simulink subsystem "Falphabeta_to_Fdq"  (R2019b)
settings: Solver=VariableStepAuto  StartTime=0.0  StopTime=10.0  RelTol=1e-3
settings Model: Creator=Nathan Petersen  LastModifiedBy=Nathan Petersen

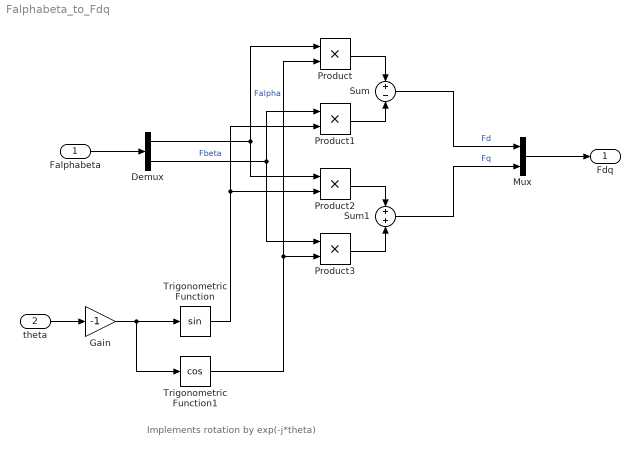
== system Falphabeta_to_Fdq ==
  note: Implements rotation by exp(-j*theta)
  Falphabeta : Inport  PortDimensions=2
  theta : Inport  Port=2  PortDimensions=1
  Demux : Demux  Outputs=2
  Gain : Gain  Gain=-1
  Mux : Mux  Inputs=2
  Product{,1..3} (4 alike) : Product
  Sum : Sum  Inputs=+-
  Sum1 : Sum
  Trigonometric Function : Trigonometry
  Trigonometric Function1 : Trigonometry  Operator=cos
  Fdq : Outport  PortDimensions=2
  wires:
  Falphabeta/1 -> Demux/1
  Product1/1 -> Sum/2
  theta/1 -> Gain/1
  Product3/1 -> Sum1/2
  Sum/1 -> Mux/1  "Fd"
  Demux/2 -> Product1/1, Product3/1  "Fbeta"
  Demux/1 -> Product2/1, Product/1  "Falpha"
  Mux/1 -> Fdq/1
  Sum1/1 -> Mux/2  "Fq"
  Product/1 -> Sum/1
  Trigonometric Function1/1 -> Product/2, Product3/2
  Product2/1 -> Sum1/1
  Trigonometric Function/1 -> Product1/2, Product2/2
  Gain/1 -> Trigonometric Function/1, Trigonometric Function1/1
